simulink model "deney4_2"  (R2025b)
settings: Solver=VariableStepAuto  StartTime=0.0  StopTime=1  RelTol=1e-3
settings Model: Creator=Seyma  LastModifiedBy=Seyma

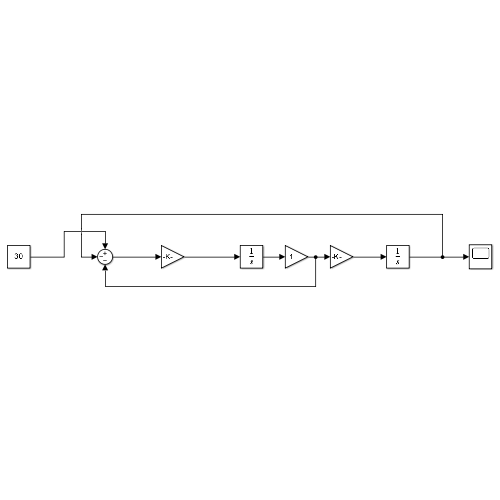
[thumbnail: Simulink's stored preview of the top-level diagram]
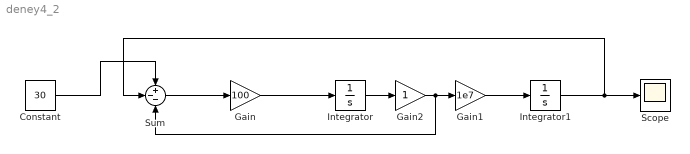
== system deney4_2 ==
  Constant : Constant  Value=30
  Gain : Gain  Gain=100
  Gain1 : Gain  Gain=1e7
  Gain2 : Gain
  Integrator : Integrator
  Integrator1 : Integrator
  Scope : Scope
      settings: ActiveDisplayYMinimum=-7.1850541237616934  ActiveDisplayYMaximum=64.665487113855249
  Sum : Sum  Inputs=+--
  wires:
  Constant/1 -> Sum/1
  Sum/1 -> Gain/1
  Gain/1 -> Integrator/1
  Gain1/1 -> Integrator1/1
  Integrator1/1 -> Sum/2, Scope/1
  Integrator/1 -> Gain2/1
  Gain2/1 -> Sum/3, Gain1/1
